simulink model "state_feedback_with_obsever"  (R2016a)
settings: Solver=VariableStepAuto  StartTime=0.0  StopTime=.15  RelTol=1e-5
undefined symbols (not defined in the file or in its folder): A, B, C, K, Ko
settings Model: Creator=manuel  LastModifiedBy=manuel

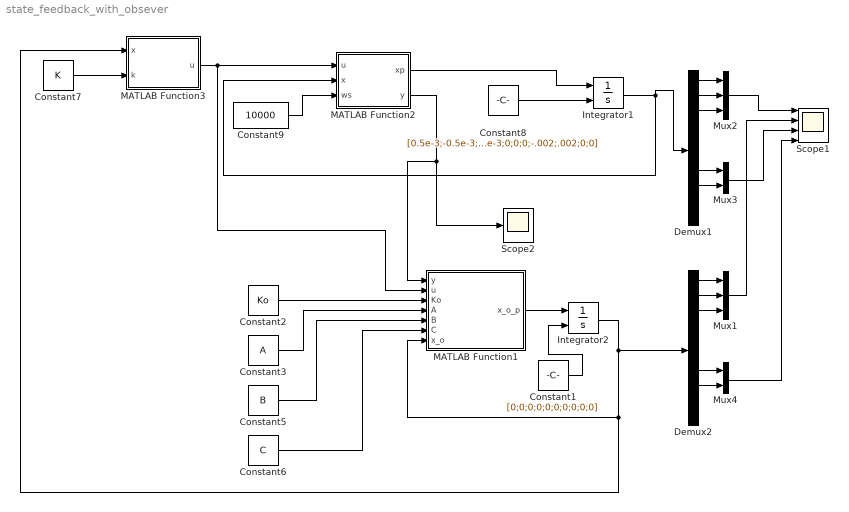
== system state_feedback_with_obsever ==
  Constant1 : Constant  Value=[0;0;0;0;0;0;0;0;0;0]
  Constant2 : Constant  Value=Ko  VectorParams1D=off
  Constant3 : Constant  Value=A  VectorParams1D=off
  Constant5 : Constant  Value=B  VectorParams1D=off
  Constant6 : Constant  Value=C  VectorParams1D=off
  Constant7 : Constant  Value=K  VectorParams1D=off
  Constant8 : Constant  Value=[0.5e-3;-0.5e-3;1e-3;0;0;0;-.002;.002;0;0]
  Constant9 : Constant  Value=10000  VectorParams1D=off
  Demux1 : Demux  Outputs=10
  Demux2 : Demux  Outputs=10
  Integrator1 : Integrator  InitialConditionSource=external
  Integrator2 : Integrator  InitialConditionSource=external
  MATLAB Function1 : MATLAB Function  TreatAsAtomicUnit=on
  MATLAB Function2 : MATLAB Function  TreatAsAtomicUnit=on
  MATLAB Function3 : MATLAB Function  TreatAsAtomicUnit=on
  Mux1 : Mux  Inputs=3
  Mux2 : Mux  Inputs=3
  Mux3 : Mux  Inputs=2
  Mux4 : Mux  Inputs=2
  Scope1 : Scope  NumInputPorts=4
  Scope2 : Scope
  wires:
  Constant8/1 -> Integrator1/2
  Integrator1/1 -> Demux1/1, MATLAB Function2/2(x)
  Constant7/1 -> MATLAB Function3/2(k)
  Demux1/1 -> Mux2/1
  Demux1/2 -> Mux2/2
  Demux1/3 -> Mux2/3
  Mux2/1 -> Scope1/1
  Demux1/7 -> Mux3/1
  Demux1/8 -> Mux3/2
  MATLAB Function2/1(xp) -> Integrator1/1
  MATLAB Function2/2(y) -> MATLAB Function1/1(y), Scope2/1
  Constant1/1 -> Integrator2/2
  MATLAB Function1/1(x_o_p) -> Integrator2/1
  Constant2/1 -> MATLAB Function1/3(Ko)
  Constant3/1 -> MATLAB Function1/4(A)
  Constant5/1 -> MATLAB Function1/5(B)
  Constant6/1 -> MATLAB Function1/6(C)
  Mux3/1 -> Scope1/3
  Integrator2/1 -> Demux2/1, MATLAB Function3/1(x), MATLAB Function1/7(x_o)
  Demux2/1 -> Mux1/1
  Demux2/2 -> Mux1/2
  Demux2/3 -> Mux1/3
  Mux1/1 -> Scope1/2
  Demux2/7 -> Mux4/1
  Demux2/8 -> Mux4/2
  Mux4/1 -> Scope1/4
  MATLAB Function3/1(u) -> MATLAB Function1/2(u), MATLAB Function2/1(u)
  Constant9/1 -> MATLAB Function2/3(ws)

== matlab function state_feedback_with_obsever/MATLAB Function1 ==
  data: y input; u input; x_o_p output; Ko input; A input; B input; C input; x_o input
function x_o_p = state_obsever(y,u,Ko,A,B,C,x_o)
%#codegen
x_o_p = A*x_o + B*u + Ko*(y-C*x_o);

== matlab function state_feedback_with_obsever/MATLAB Function2 ==
  data: u input; x input; xp output; y output; ws input
function [xp,y] = fcn(u,x,ws)

Fd_x = 0;
Fd_y = 0;
Fd_z = 0;
Md_y = 0;
Md_z = 0;
[xp,y] = hmb_non_linear_model(x,u,ws,Fd_x,Fd_y,Fd_z,Md_y,Md_z);

end

== matlab function state_feedback_with_obsever/MATLAB Function3 ==
  data: x input; k input; u output
function u = feedback_controller(x,k)
%#codegen
u = -k*x;
